simulink model "Racing_2019"  (R2017a)
settings: Solver=FixedStepDiscrete  StartTime=0.0  StopTime=Inf  FixedStep=1e-3  RelTol=1e-3  EnableMultiTasking=on
PostLoadFcn:
  | , if any(exist('dsrtsu_mdlpostloadfcn', 'file') == [2, 3, 6]), try dsrtsu_mdlpostloadfcn('Execute', bdroot); catch fprintf('Error in PostLoadFcn (dsrtsu_mdlpostloadfcn) for model "%s":\n %s\n', bdroot, lasterr); end, end,
undefined symbols (not defined in the file): Accu_Fans_Enable, Accu_Fans_ON, Accu_Fans_PWM, APPS_Bypass, APPS_Value, AUX_Error_Time, Batt_Temp_High_Threshold, Batt_Temp_Low_Threshold, BMS_Error_Time, BMS_Reset, BMS_Reset_Enable, BMS_Status_Bypass, Brake_Plausibility_Threshold, Brake_Threshold, Brakelight_Test, Braking_Torque, BSPD_State_Bypass, Buzzer, Buzzer_Silent, Buzzer_Test, Calibrate, CAN_Rx_FMEA_Enable, CAN_Status_FMEA_Enable, CAN_Tx_FMEA_Enable, Car_Reset, Car_Reset_Enable, Dash_Fan_PWM, DiscIntNeverNeededParam, DRS_Enable, DRS_PWM_OFF, DRS_PWM_ON, ED_Enable, ED_On, Eject_USB, Enable_Kill, Enable_LED_Test, Fans_Left_Enable, Fans_Left_ON, Fans_Left_PWM, Fans_Right_Enable, Fans_Right_ON, Fans_Right_PWM, I_MAX, IGBT_Temp_High_Threshold, IGBT_Temp_Low_Threshold, Inverter_CAN_Tx_Enable, Inverter_Frequency, KW_Max_Regen_Reset, KW_Max_Reset, LV_DCDC_Temp_High_Threshold, LV_DCDC_Temp_Low_Threshold, magnitude, Plausibility_Bypass, Power_Limiter_Killswitch, Power_Target_kW, Pump_Left_Enable, Pump_Left_ON, Pump_Right_Enable, Pump_Right_ON, Pump_Signal_Left ... (+13)
libraries: rtiusbflightreclib x206, simulink x153, rtican x52, powerlib_meascontrol x47, simulink_extras x17, rti1401lib_adc_type4 x6, rti1401lib_dio_type4 x3, rti1401lib_II_base x1
(part 14 of 23)

== system Racing_2019/Inverters CAN Tx ==
  note: Error = 0
  Torque Right : Inport
  Torque Left : Inport  Port=2
  10Hz Pulse : DiscretePulseGenerator  Period=100  SampleTime=0.001
  Add : Sum
  Add1 : Sum
  Add2 : Sum
  Bus Creator : BusCreator  Inputs='Mode','ID','Time'
  Bus Selector : BusSelector  OutputSignals=Mode
  Bus Selector1 : BusSelector  OutputSignals=ID,ID,ID
  Bus Selector2 : BusSelector  OutputSignals=Time,Time,Time
  Bus Selector3 : BusSelector  OutputSignals=Mode
  Bus Selector4 : BusSelector  OutputSignals=ID,ID,ID
  Bus Selector5 : BusSelector  OutputSignals=Time,Time,Time
  Bus Selector6 : BusSelector  OutputSignals=Time
  Bus Selector7 : BusSelector  OutputSignals=ID
  Bus Selector8 : BusSelector  OutputSignals=Time
  Bus Selector9 : BusSelector  OutputSignals=ID
  Constant : Constant  Value=I_MAX
  Constant1 : Constant  Value=Inverter_CAN_Tx_Enable
  Constant2 : Constant  Value=Set_Inverter_Settings
  Constant3 : Constant  Value=Set_ID
  Constant4 : Constant  Value=0
  Constant5 : Constant  Value=0
  Constant6 : Constant  Value=RPM_MAX
  Data Type Conversion{,1..2,5..6} (5 alike) : DataTypeConversion  OutDataTypeStr=double
  Data Type Conversion3 : DataTypeConversion  OutDataTypeStr=uint8
  Data Type Conversion4 : DataTypeConversion  OutDataTypeStr=uint8
  Data Type Conversion7 : DataTypeConversion  OutDataTypeStr=uint16
  Data Type Conversion8 : DataTypeConversion  OutDataTypeStr=uint16
  Data Type Conversion9 : DataTypeConversion  OutDataTypeStr=uint16
  Delay 50ms : Delay  DelayLength=50  SampleTime=0.001
  Edge Detector : powerlib_meascontrol/Logic/Edge Detector  model=Rising  ic=0  Ts=-1
      settings: SourceProductName=Simscape Power Systems  SourceProductBaseCode=PS
  Edge Detector1 : powerlib_meascontrol/Logic/Edge Detector  model=Rising  ic=0  Ts=-1
      settings: SourceProductName=Simscape Power Systems  SourceProductBaseCode=PS
  Gain_Left : Gain  Gain=-32767/1000
  Gain_Right : Gain  Gain=-32767/1000
  Inverter_LEFT_CAN_0x161 : Delay  DelayLength=1000  InitialCondition=1  ExternalReset=Level
      settings: InputPortMap=u0,r5
  Inverter_LEFT_CAN_Tx_Counter : Memory  InheritSampleTime=on
  Inverter_Left_CAN_Tx : rtican/RTICAN Transmit (TX)   Reserved1=[]  Reserved2=[]  Reserved3=[]  Reserved4=[]  SfcnMessage=[]  Msg_Struct=[]  BoardTypeNo=[]  BoardNo=[]  ChannelNo=[]  Parameters=[]  DialogFcn=[]  UnitName=[]  Revision=[]  UnitValues=[]  DSProperties=struct('RTI',struct('Version',uint32(5),'BlockType',struct('isSLSource',uint8(1),'isSLSink',uint8(1),'isHWSource',uint8(0),'isHWSink',uint8(0),'isSetup',uint8(0),'isInline',uint8(1),'isNonInline',uint8(0),'isInterrupt',uint8(0),'isChannelwise',uint8(0)),'IOBoardType','RTICAN','UnitType','MESSAGE','Identifier','TX','DialogType','MSVC','BlockSet','RTICAN','SlaveProcessor','CAN'))  RTIBlockInterface=struct('InputPortsWidth',int32([1 1 1 1 1 1 1 1 1 1]),'InputPortsActive',[1 1 1 1 1 1 1 1 1 1],'InputPortsName',{{'REGID_Mode','REGID','b1_77','b1_78','Torque_CMD','b1_200','Time','b2_77','b2_78','b2_200'}},'InputPortsDataType',{{'SS_DOUBLE','SS_DOUBLE','SS_DOUBLE','SS_DOUBLE','SS_DOUBLE','SS_DOUBLE','SS_DOUBLE','SS_DOUBLE','SS_DOUBLE','SS_DOUBLE'}},'OutputPortsWidth',int32(1),'OutputPortsActive',1,'OutputPortsName',{{['TX status']}},'DialogFcn','rtican_message_interface_gui','BlockDisplay',{{'','center'}},'IconTransparency','on','InitLevel',3,'BlockName',struct('Token',{{'Inverter_Left_CAN_Tx'}}),'SampleTime',{{0.001}},'TriggerPort',{{'none'}},'EnablePort',{{'yes'}})  RTIBlockParameters=struct('BoardTypeNo',{{1,'OFF',[]}},'BoardNo',{{1,'ON',[1 16]}},'ChannelNo',{{1,'ON',[1 2]}},'Parameters',{{struct('DataFileSupport',struct('DataFileSelectedMaster',0,'DataFileSelectedLocal',0,'DataFileName',['<no datafile support>|'],'DataFileDate','','SelectedFile',['<no file selected>']),'Options',struct('StatusSelected',1,'TimeSelected',0,'DeltaTimeSelected',0,'DelayTimeSelected',0,'DelayTimeTXCommandSelected',0,'EncodeSetUnusedBitsToOne',0,'EnableMsgLoopback',0,'TriggerPort',struct('Selected',0,'TriggerType',0),'EnablePortSelected',1,'SignalOnPortnameSelected',1,'UserCoding',struct('Selected',0,'InterfaceFile','UserEncodingFile','FcnName','UserEncodeFcn','InportSelected',0,'InportWidth',1,'OutportSelected',0,'OutportWidth',1),'TerminationMsg',struct('Selected',0,'Byte0_7','0'),'InitialMsg',struct('Selected',0,'Byte0_7','0')),'Message',struct('MsgOnBlocknameSelected',1,'MsgName','Inverter_Left_CAN_Tx','MsgIdFormat',0,'MsgId',353,'MsgLength',3,'NumSignals',10,'SampleTime',0.001,'StartTime',struct('Selected',0,'Value',9),'AutoRepeatTime',struct('Selected',0,'Value',0.1),'Timeout',struct('Selected',0,'Value',0.1),'DelayTime',struct('Selected',0,'Value',0.1),'Signal',struct('SgnName',{'REGID_Mode','REGID','b1_77','b1_78','Torque_CMD','b1_200','Time','b2_77','b2_78','b2_200'},'SgnStartBit',{0,8,8,8,8,8,16,16,16,16},'SgnLength',{8,8,8,8,16,8,8,8,8,8},'SgnType',{1,2,2,2,2,2,2,2,2,2},'ModeValue',{-1,61,77,78,144,200,61,77,78,200},'DataType',{0,0,0,0,1,0,0,0,0,0},'ByteLayout',{0,0,0,0,0,0,0,0,0,0},'Factor',{1,1,1,1,1,1,1,1,1,1},'Offset',{0,0,0,0,0,0,0,0,0,0},'SgnComment',{{''},{''},{''},{''},{''},{''},{''},{''},{''},{''}},'SgnUnit',{'','','','','','','','','',''},'Min',{0,0,0,0,0,0,0,0,0,0},'Max',{255,255,255,255,255,0,255,255,255,0},'SLDataType',{'SS_DOUBLE','SS_DOUBLE','SS_DOUBLE','SS_DOUBLE','SS_DOUBLE','SS_DOUBLE','SS_DOUBLE','SS_DOUBLE','SS_DOUBLE','SS_DOUBLE'}),'MsgIdNumFormat',1,'MsgComment',{{''}}),'Version',1.2,'general',struct('isFromLib',0)),'OFF',[]}},'GroupId',{{struct('Group',{{'RTICAN'}},'No',1,'Behavior',{{'NAMECHANGE'}},'BlockType',{{'SINK'}},'NameChangeFlag',0),'OFF',[]}},'SFcnRTICANMessage',{{struct('MsgType','TX','SFcnPortType','Scalar','MsgName','Inverter_Left_CAN_Tx','MsgIdFormat','STD','MsgId',353,'MsgLength',3,'NumSignals',10,'SampleTime',0.001,'StartTime',struct('Selected','no','Value',9),'AutoRepeatTime',struct('Selected','no','Value',0.1),'Timeout',struct('Selected','no','Value',0.1),'Signal',struct('SgnName',{'REGID_Mode','REGID','b1_77','b1_78','Torque_CMD','b1_200','Time','b2_77','b2_78','b2_200'},'SgnStartBit',{0,8,8,8,8,8,16,16,16,16},'SgnLength',{8,8,8,8,16,8,8,8,8,8},'SgnType',{'mode','mode-dependent','mode-dependent','mode-dependent','mode-dependent','mode-dependent','mode-dependent','mode-dependent','mode-dependent','mode-dependent'},'ModeValue',{-1,61,77,78,144,200,61,77,78,200},'DataType',{['unsigned int'],['unsigned int'],['unsigned int'],['unsigned int'],['signed int'],['unsigned int'],['unsigned int'],['unsigned int'],['unsigned int'],['unsigned int']},'ByteLayout',{['little endian'],['little endian'],['little endian'],['little endian'],['little endian'],['little endian'],['little endian'],['little endian'],['little endian'],['little endian']},'Factor',{1,1,1,1,1,1,1,1,1,1},'Offset',{0,0,0,0,0,0,0,0,0,0},'SLDataType',{'SS_DOUBLE','SS_DOUBLE','SS_DOUBLE','SS_DOUBLE','SS_DOUBLE','SS_DOUBLE','SS_DOUBLE','SS_DOUBLE','SS_DOUBLE','SS_DOUBLE'}),'StatusSelected','yes','TimeSelected','no','DeltaTimeSelected','no','DelayTimeSelected','no','DelayTimeTXCommandSelected','no','EncodeSetUnusedBitsToOne','no','EnableMsgLoopback','no','TriggerPort',struct('Selected','no','TriggerType',0),'EnablePortSelected','yes','UserCoding',struct('Selected','no','InterfaceFile','UserEncodingFile','FcnName','UserEncodeFcn','InportSelected','no','InportWidth',1,'OutportSelected','no','OutportWidth',1),'TerminationMsg',struct('Selected','no','Byte0','0x00','Byte1','0x00','Byte2','0x00','Byte3','0x00','Byte4','0x00','Byte5','0x00','Byte6','0x00','Byte7','0x00'),'InitialMsg',struct('Selected','no','Byte0','0x00','Byte1','0x00','Byte2','0x00','Byte3','0x00','Byte4','0x00','Byte5','0x00','Byte6','0x00','Byte7','0x00'),'BoardType','DS1','BoardNo',1,'ControllerNo',1),'OFF',[]}},'TLCFileName',{{'rtican_tx_message','OFF',[]}})  RTISFcnParameters=struct('SFcnRTICANMessage','struct','TLCFileName','char')  RTIBlockParaDefault=struct('BoardTypeNo',4302,'BoardNo',1,'ChannelNo',1,'Parameters',struct('DataFileSupport',struct('DataFileSelectedMaster',0,'DataFileSelectedLocal',0,'DataFileName','','DataFileDate','','SelectedFile',['<no file selected>']),'Options',struct('StatusSelected',1,'TimeSelected',1,'DeltaTimeSelected',1,'DelayTimeSelected',1,'DelayTimeTXCommandSelected',0,'EncodeSetUnusedBitsToOne',0,'EnableMsgLoopback',0,'TriggerPort',struct('Selected',0,'TriggerType','rising'),'EnablePortSelected',0,'SignalOnPortnameSelected',1,'UserCoding',struct('Selected',0,'InterfaceFile','UserEncodingFile','FcnName','UserEncodeFcn','InportSelected',0,'InportWidth',1,'OutportSelected',0,'OutportWidth',1),'TerminationMsg',struct('Selected',0,'Byte0_7','0'),'InitialMsg',struct('Selected',0,'Byte0_7','0')),'Message',struct('MsgOnBlocknameSelected',0,'MsgName',['TX Message'],'MsgIdFormat',0,'MsgId',100,'MsgLength',8,'NumSignals',1,'SampleTime',-1,'StartTime',struct('Selected',0,'Value',0),'AutoRepeatTime',struct('Selected',0,'Value',0.1),'Timeout',struct('Selected',0,'Value',0.1),'DelayTime',struct('Selected',0,'Value',0.1),'Signal',struct('SgnName',['TX signal'],'SgnStartBit',0,'SgnLength',8,'SgnType',0,'ModeValue',-1,'DataType',0,'SLDataType','SS_DOUBLE','ByteLayout',0,'Factor',1,'Offset',0,'Min',0,'Max',255,'SgnComment',{{}},'SgnUnit',''),'MsgIdNumFormat',0,'MsgComment',{{''}}),'Version',1.2,'general',struct('isFromLib',1)),'GroupId',struct('Group',{{'RTICAN'}},'No',1,'Behavior',{{'NAMECHANGE'}},'BlockType',{{'SINK'}},'NameChangeFlag',0),'SFcnRTICANMessage',struct('MsgType','TX','MsgName',['TX Message'],'MsgIdFormat','STD','MsgId',100,'MsgLength',2,'NumSignals',1,'SampleTime',-1,'StartTime',struct('Selected','no','Value',0),'AutoRepeatTime',struct('Selected','no','Value',0.1),'Timeout',struct('Selected','no','Value',0.1),'DelayTime',struct('Selected','no','Value',0.1),'Signal',struct('SgnName',['TX signal'],'SgnStartBit',0,'SgnLength',8,'SgnType','standard','ModeValue',-1,'DataType',['unsigned int'],'ByteLayout',['little endian'],'SLDataType','SS_DOUBLE','Factor',1,'Offset',0),'StatusSelected','yes','TimeSelected','yes','DeltaTimeSelected','yes','DelayTimeSelected','yes','EnablePortSelected','no','EnableMsgLoopback','no','DelayTimeTXCommandSelected','no','EncodeSetUnusedBitsToOne','no','UserCoding',struct('Selected','no','InterfaceFile','UserDecodingFile','FcnName','UserDecodeFcn','InportSelected','no','InportWidth',1,'OutportSelected','no','OutportWidth',1),'TerminationMsg',struct('Selected','no','Byte0','0x00','Byte1','0x00','Byte2','0x00','Byte3','0x00','Byte4','0x00','Byte5','0x00','Byte6','0x00','Byte7','0x00'),'InitialMsg',struct('Selected','no','Byte0','0x00','Byte1','0x00','Byte2','0x00','Byte3','0x00','Byte4','0x00','Byte5','0x00','Byte6','0x00','Byte7','0x00'),'TriggerPort',struct('Selected','no','TriggerType','rising'),'BoardType','DS4302','BoardNo',1,'ControllerNo',1,'SFcnPortType','Scalar'),'TLCFileName','rtican_tx_message')
      settings: AttributesFormatString=Group Id: RTICAN1\n  SourceProductName=dSPACE RTI CAN Blockset
  Inverter_RIGHT_CAN_0x162 : Delay  DelayLength=1000  InitialCondition=1  ExternalReset=Level
      settings: InputPortMap=u0,r5
  Inverter_RIGHT_CAN_Tx_Counter : Memory  InheritSampleTime=on
  Inverter_Right_CAN_Tx : rtican/RTICAN Transmit (TX)   Reserved1=[]  Reserved2=[]  Reserved3=[]  Reserved4=[]  SfcnMessage=[]  Msg_Struct=[]  BoardTypeNo=[]  BoardNo=[]  ChannelNo=[]  Parameters=[]  DialogFcn=[]  UnitName=[]  Revision=[]  UnitValues=[]  DSProperties=struct('RTI',struct('Version',uint32(5),'BlockType',struct('isSLSource',uint8(1),'isSLSink',uint8(1),'isHWSource',uint8(0),'isHWSink',uint8(0),'isSetup',uint8(0),'isInline',uint8(1),'isNonInline',uint8(0),'isInterrupt',uint8(0),'isChannelwise',uint8(0)),'IOBoardType','RTICAN','UnitType','MESSAGE','Identifier','TX','DialogType','MSVC','BlockSet','RTICAN','SlaveProcessor','CAN'))  RTIBlockInterface=struct('InputPortsWidth',int32([1 1 1 1 1 1 1 1 1 1]),'InputPortsActive',[1 1 1 1 1 1 1 1 1 1],'InputPortsName',{{'REGID_Mode','REGID','b1_77','b1_78','Torque_Value','b1_200','Time','b2_77','b2_78','b2_200'}},'InputPortsDataType',{{'SS_DOUBLE','SS_DOUBLE','SS_DOUBLE','SS_DOUBLE','SS_DOUBLE','SS_DOUBLE','SS_DOUBLE','SS_DOUBLE','SS_DOUBLE','SS_DOUBLE'}},'OutputPortsWidth',int32(1),'OutputPortsActive',1,'OutputPortsName',{{['TX status']}},'DialogFcn','rtican_message_interface_gui','BlockDisplay',{{'','center'}},'IconTransparency','on','InitLevel',3,'BlockName',struct('Token',{{'Inverter_Right_CAN_Tx'}}),'SampleTime',{{0.001}},'TriggerPort',{{'none'}},'EnablePort',{{'yes'}})  RTIBlockParameters=struct('BoardTypeNo',{{1,'OFF',[]}},'BoardNo',{{1,'ON',[1 16]}},'ChannelNo',{{2,'ON',[1 2]}},'Parameters',{{struct('DataFileSupport',struct('DataFileSelectedMaster',0,'DataFileSelectedLocal',0,'DataFileName',['<no datafile support>|'],'DataFileDate','','SelectedFile',['<no file selected>']),'Options',struct('StatusSelected',1,'TimeSelected',0,'DeltaTimeSelected',0,'DelayTimeSelected',0,'DelayTimeTXCommandSelected',0,'EncodeSetUnusedBitsToOne',0,'EnableMsgLoopback',0,'TriggerPort',struct('Selected',0,'TriggerType',0),'EnablePortSelected',1,'SignalOnPortnameSelected',1,'UserCoding',struct('Selected',0,'InterfaceFile','UserEncodingFile','FcnName','UserEncodeFcn','InportSelected',0,'InportWidth',1,'OutportSelected',0,'OutportWidth',1),'TerminationMsg',struct('Selected',0,'Byte0_7','0'),'InitialMsg',struct('Selected',0,'Byte0_7','0')),'Message',struct('MsgOnBlocknameSelected',1,'MsgName','Inverter_Right_CAN_Tx','MsgIdFormat',0,'MsgId',354,'MsgLength',3,'NumSignals',10,'SampleTime',0.001,'StartTime',struct('Selected',0,'Value',5),'AutoRepeatTime',struct('Selected',0,'Value',0.1),'Timeout',struct('Selected',0,'Value',0.1),'DelayTime',struct('Selected',0,'Value',0.1),'Signal',struct('SgnName',{'REGID_Mode','REGID','b1_77','b1_78','Torque_Value','b1_200','Time','b2_77','b2_78','b2_200'},'SgnStartBit',{0,8,8,8,8,8,16,16,16,16},'SgnLength',{8,8,8,8,16,8,8,8,8,8},'SgnType',{1,2,2,2,2,2,2,2,2,2},'ModeValue',{-1,61,77,78,144,200,61,77,78,200},'DataType',{0,0,0,0,1,0,0,0,0,0},'ByteLayout',{0,0,0,0,0,0,0,0,0,0},'Factor',{1,1,1,1,1,1,1,1,1,1},'Offset',{0,0,0,0,0,0,0,0,0,0},'SgnComment',{{''},{''},{''},{''},{''},{''},{''},{''},{''},{''}},'SgnUnit',{'','','','','','','','','',''},'Min',{0,0,0,0,0,0,0,0,0,0},'Max',{255,255,255,255,255,0,255,255,255,0},'SLDataType',{'SS_DOUBLE','SS_DOUBLE','SS_DOUBLE','SS_DOUBLE','SS_DOUBLE','SS_DOUBLE','SS_DOUBLE','SS_DOUBLE','SS_DOUBLE','SS_DOUBLE'}),'MsgIdNumFormat',1,'MsgComment',{{''}}),'Version',1.2,'general',struct('isFromLib',0)),'OFF',[]}},'GroupId',{{struct('Group',{{'RTICAN'}},'No',2,'Behavior',{{'NAMECHANGE'}},'BlockType',{{'SINK'}},'NameChangeFlag',0),'OFF',[]}},'SFcnRTICANMessage',{{struct('MsgType','TX','SFcnPortType','Scalar','MsgName','Inverter_Right_CAN_Tx','MsgIdFormat','STD','MsgId',354,'MsgLength',3,'NumSignals',10,'SampleTime',0.001,'StartTime',struct('Selected','no','Value',5),'AutoRepeatTime',struct('Selected','no','Value',0.1),'Timeout',struct('Selected','no','Value',0.1),'Signal',struct('SgnName',{'REGID_Mode','REGID','b1_77','b1_78','Torque_Value','b1_200','Time','b2_77','b2_78','b2_200'},'SgnStartBit',{0,8,8,8,8,8,16,16,16,16},'SgnLength',{8,8,8,8,16,8,8,8,8,8},'SgnType',{'mode','mode-dependent','mode-dependent','mode-dependent','mode-dependent','mode-dependent','mode-dependent','mode-dependent','mode-dependent','mode-dependent'},'ModeValue',{-1,61,77,78,144,200,61,77,78,200},'DataType',{['unsigned int'],['unsigned int'],['unsigned int'],['unsigned int'],['signed int'],['unsigned int'],['unsigned int'],['unsigned int'],['unsigned int'],['unsigned int']},'ByteLayout',{['little endian'],['little endian'],['little endian'],['little endian'],['little endian'],['little endian'],['little endian'],['little endian'],['little endian'],['little endian']},'Factor',{1,1,1,1,1,1,1,1,1,1},'Offset',{0,0,0,0,0,0,0,0,0,0},'SLDataType',{'SS_DOUBLE','SS_DOUBLE','SS_DOUBLE','SS_DOUBLE','SS_DOUBLE','SS_DOUBLE','SS_DOUBLE','SS_DOUBLE','SS_DOUBLE','SS_DOUBLE'}),'StatusSelected','yes','TimeSelected','no','DeltaTimeSelected','no','DelayTimeSelected','no','DelayTimeTXCommandSelected','no','EncodeSetUnusedBitsToOne','no','EnableMsgLoopback','no','TriggerPort',struct('Selected','no','TriggerType',0),'EnablePortSelected','yes','UserCoding',struct('Selected','no','InterfaceFile','UserEncodingFile','FcnName','UserEncodeFcn','InportSelected','no','InportWidth',1,'OutportSelected','no','OutportWidth',1),'TerminationMsg',struct('Selected','no','Byte0','0x00','Byte1','0x00','Byte2','0x00','Byte3','0x00','Byte4','0x00','Byte5','0x00','Byte6','0x00','Byte7','0x00'),'InitialMsg',struct('Selected','no','Byte0','0x00','Byte1','0x00','Byte2','0x00','Byte3','0x00','Byte4','0x00','Byte5','0x00','Byte6','0x00','Byte7','0x00'),'BoardType','DS1','BoardNo',1,'ControllerNo',2),'OFF',[]}},'TLCFileName',{{'rtican_tx_message','OFF',[]}})  RTISFcnParameters=struct('SFcnRTICANMessage','struct','TLCFileName','char')  RTIBlockParaDefault=struct('BoardTypeNo',4302,'BoardNo',1,'ChannelNo',1,'Parameters',struct('DataFileSupport',struct('DataFileSelectedMaster',0,'DataFileSelectedLocal',0,'DataFileName','','DataFileDate','','SelectedFile',['<no file selected>']),'Options',struct('StatusSelected',1,'TimeSelected',1,'DeltaTimeSelected',1,'DelayTimeSelected',1,'DelayTimeTXCommandSelected',0,'EncodeSetUnusedBitsToOne',0,'EnableMsgLoopback',0,'TriggerPort',struct('Selected',0,'TriggerType','rising'),'EnablePortSelected',0,'SignalOnPortnameSelected',1,'UserCoding',struct('Selected',0,'InterfaceFile','UserEncodingFile','FcnName','UserEncodeFcn','InportSelected',0,'InportWidth',1,'OutportSelected',0,'OutportWidth',1),'TerminationMsg',struct('Selected',0,'Byte0_7','0'),'InitialMsg',struct('Selected',0,'Byte0_7','0')),'Message',struct('MsgOnBlocknameSelected',0,'MsgName',['TX Message'],'MsgIdFormat',0,'MsgId',100,'MsgLength',8,'NumSignals',1,'SampleTime',-1,'StartTime',struct('Selected',0,'Value',0),'AutoRepeatTime',struct('Selected',0,'Value',0.1),'Timeout',struct('Selected',0,'Value',0.1),'DelayTime',struct('Selected',0,'Value',0.1),'Signal',struct('SgnName',['TX signal'],'SgnStartBit',0,'SgnLength',8,'SgnType',0,'ModeValue',-1,'DataType',0,'SLDataType','SS_DOUBLE','ByteLayout',0,'Factor',1,'Offset',0,'Min',0,'Max',255,'SgnComment',{{}},'SgnUnit',''),'MsgIdNumFormat',0,'MsgComment',{{''}}),'Version',1.2,'general',struct('isFromLib',1)),'GroupId',struct('Group',{{'RTICAN'}},'No',1,'Behavior',{{'NAMECHANGE'}},'BlockType',{{'SINK'}},'NameChangeFlag',0),'SFcnRTICANMessage',struct('MsgType','TX','MsgName',['TX Message'],'MsgIdFormat','STD','MsgId',100,'MsgLength',2,'NumSignals',1,'SampleTime',-1,'StartTime',struct('Selected','no','Value',0),'AutoRepeatTime',struct('Selected','no','Value',0.1),'Timeout',struct('Selected','no','Value',0.1),'DelayTime',struct('Selected','no','Value',0.1),'Signal',struct('SgnName',['TX signal'],'SgnStartBit',0,'SgnLength',8,'SgnType','standard','ModeValue',-1,'DataType',['unsigned int'],'ByteLayout',['little endian'],'SLDataType','SS_DOUBLE','Factor',1,'Offset',0),'StatusSelected','yes','TimeSelected','yes','DeltaTimeSelected','yes','DelayTimeSelected','yes','EnablePortSelected','no','EnableMsgLoopback','no','DelayTimeTXCommandSelected','no','EncodeSetUnusedBitsToOne','no','UserCoding',struct('Selected','no','InterfaceFile','UserDecodingFile','FcnName','UserDecodeFcn','InportSelected','no','InportWidth',1,'OutportSelected','no','OutportWidth',1),'TerminationMsg',struct('Selected','no','Byte0','0x00','Byte1','0x00','Byte2','0x00','Byte3','0x00','Byte4','0x00','Byte5','0x00','Byte6','0x00','Byte7','0x00'),'InitialMsg',struct('Selected','no','Byte0','0x00','Byte1','0x00','Byte2','0x00','Byte3','0x00','Byte4','0x00','Byte5','0x00','Byte6','0x00','Byte7','0x00'),'TriggerPort',struct('Selected','no','TriggerType','rising'),'BoardType','DS4302','BoardNo',1,'ControllerNo',1,'SFcnPortType','Scalar'),'TLCFileName','rtican_tx_message')
      settings: AttributesFormatString=Group Id: RTICAN2\n  SourceProductName=dSPACE RTI CAN Blockset
  Inverters CAN Send : MATLAB Function  TreatAsAtomicUnit=on
  Logical Operator : Logic  Inputs=3  AllPortsSameDT=off  OutDataTypeStr=boolean
  Logical Operator1 : Logic  Operator=NOT  AllPortsSameDT=off  OutDataTypeStr=boolean
  Logical Operator2 : Logic  AllPortsSameDT=off  OutDataTypeStr=boolean
  Memory : Memory  X0=-14
  Switch : Switch  Criteria=u2 > Threshold
  Switch1 : Switch  Criteria=u2 > Threshold
  Torque AND : Logic  AllPortsSameDT=off  OutDataTypeStr=boolean
  Torque Mode : simulink/Logic and Bit Operations/Compare To Constant  relop===  const=144  OutDataTypeStr=boolean
  USB_Torque_Left : rtiusbflightreclib/USB_FLIGHT_REC_BL1  VarName=Torque_Left  DataType=UInt16  SampleTime=-1  TLCFileName=rtiusbflightrecwrite  Reserved1=[]  Reserved2=[]  Reserved3=[]  Reserved4=[]  DSProperties=struct('RTI',struct('Version',uint32(3),'BlockType',struct('isSLSource',uint8(0),'isSLSink',uint8(1),'isHWSource',uint8(0),'isHWSink',uint8(0),'isSetup',uint8(0),'isInline',uint8(1),'isNonInline',uint8(0),'isInterrupt',uint8(0),'isChannelwise',uint8(0)),'IOBoardType',{{'DSUSB','FLIGHTREC'}},'UnitType','FLIGHTREC','Identifier','WRITE','DialogType','SL','BlockSet','RTIUSBFLIGHTREC','SlaveProcessor','NONE'))  RTIBlockInterface=struct('InputPortsActive',1,'InputPortsWidth',int32(1),'InputPortsDataType',{{'SS_UINT16'}},'BlockDisplay',{{['Write to\nUSB Flight Recorder'],'center'}},'IconTransparency','off','InitLevel',3,'BlockName',struct('Token',{{'USB_FLIGHT_REC_BL1'}}),'MaskDescription',['Write input to the Flight Recorder. Recorded data can be referenced by the specified variable.'],'SampleTime',{{-1}})  RTIBlockParameters=struct('VarName',{{'Torque_Left','OFF',[]}},'DataType',{{'UInt16','OFF',[]}},'SampleTime',{{-1,'OFF',[]}},'TLCFileName',{{'rtiusbflightrecwrite','OFF',[]}})  RTISFcnParameters=struct('VarName','char','DataType','char','SampleTime','double','TLCFileName','char')  RTIBlockParaDefault=struct('VarName','Var1','DataType','Single','SampleTime',-1,'TLCFileName','rtiusbflightrecwrite')
      settings: SourceProductName=dSPACE RTI USB Flight Rec Blockset
  USB_Torque_Right : rtiusbflightreclib/USB_FLIGHT_REC_BL1  VarName=Torque_Right  DataType=UInt16  SampleTime=-1  TLCFileName=rtiusbflightrecwrite  Reserved1=[]  Reserved2=[]  Reserved3=[]  Reserved4=[]  DSProperties=struct('RTI',struct('Version',uint32(3),'BlockType',struct('isSLSource',uint8(0),'isSLSink',uint8(1),'isHWSource',uint8(0),'isHWSink',uint8(0),'isSetup',uint8(0),'isInline',uint8(1),'isNonInline',uint8(0),'isInterrupt',uint8(0),'isChannelwise',uint8(0)),'IOBoardType',{{'DSUSB','FLIGHTREC'}},'UnitType','FLIGHTREC','Identifier','WRITE','DialogType','SL','BlockSet','RTIUSBFLIGHTREC','SlaveProcessor','NONE'))  RTIBlockInterface=struct('InputPortsActive',1,'InputPortsWidth',int32(1),'InputPortsDataType',{{'SS_UINT16'}},'BlockDisplay',{{['Write to\nUSB Flight Recorder'],'center'}},'IconTransparency','off','InitLevel',3,'BlockName',struct('Token',{{'USB_FLIGHT_REC_BL1'}}),'MaskDescription',['Write input to the Flight Recorder. Recorded data can be referenced by the specified variable.'],'SampleTime',{{-1}})  RTIBlockParameters=struct('VarName',{{'Torque_Right','OFF',[]}},'DataType',{{'UInt16','OFF',[]}},'SampleTime',{{-1,'OFF',[]}},'TLCFileName',{{'rtiusbflightrecwrite','OFF',[]}})  RTISFcnParameters=struct('VarName','char','DataType','char','SampleTime','double','TLCFileName','char')  RTIBlockParaDefault=struct('VarName','Var1','DataType','Single','SampleTime',-1,'TLCFileName','rtiusbflightrecwrite')
      settings: SourceProductName=dSPACE RTI USB Flight Rec Blockset
  "Torque CAN " : Outport
  wires:
  Inverters CAN Send/1(Mode) -> Data Type Conversion/1
  Inverters CAN Send/2(ID) -> Data Type Conversion1/1
  Inverters CAN Send/3(Time) -> Data Type Conversion2/1
  Data Type Conversion/1 -> Torque Mode/1, Bus Creator/1  "Mode"
  Data Type Conversion1/1 -> Bus Creator/2  "ID"
  Data Type Conversion2/1 -> Bus Creator/3  "Time"
  Bus Selector/1 -> Inverter_Right_CAN_Tx/1  "<Mode>"
  Bus Selector1/1 -> Inverter_Right_CAN_Tx/2  "<ID>"
  Bus Selector1/2 -> Inverter_Right_CAN_Tx/3  "<ID>"
  Bus Selector1/3 -> Inverter_Right_CAN_Tx/4  "<ID>"
  Bus Selector2/1 -> Inverter_Right_CAN_Tx/7  "<Time>"
  Bus Selector2/2 -> Inverter_Right_CAN_Tx/8  "<Time>"
  Bus Selector2/3 -> Inverter_Right_CAN_Tx/9  "<Time>"
  Bus Selector4/3 -> Inverter_Left_CAN_Tx/4  "<ID>"
  Bus Selector5/3 -> Inverter_Left_CAN_Tx/9  "<Time>"
  Bus Selector3/1 -> Inverter_Left_CAN_Tx/1  "<Mode>"
  Bus Creator/1 -> Bus Selector7/1, Bus Selector/1, Bus Selector1/1, Bus Selector2/1, Bus Selector6/1, Bus Selector9/1, Bus Selector8/1, Bus Selector5/1, Bus Selector4/1, Bus Selector3/1
  Bus Selector4/1 -> Inverter_Left_CAN_Tx/2  "<ID>"
  Bus Selector5/1 -> Inverter_Left_CAN_Tx/7  "<Time>"
  Bus Selector4/2 -> Inverter_Left_CAN_Tx/3  "<ID>"
  Bus Selector5/2 -> Inverter_Left_CAN_Tx/8  "<Time>"
  Constant/1 -> Inverters CAN Send/2(Icont)
  Torque Mode/1 -> Logical Operator/1, Switch/2, Logical Operator1/1, Switch/1
  Delay 50ms/1 -> Switch/3
  Switch/1 -> Torque AND/2
  Constant1/1 -> Torque AND/1
  10Hz Pulse/1 -> Logical Operator2/1, Delay 50ms/1
  Logical Operator2/1 -> Data Type Conversion7/1
  Add/1 -> Memory/1
  Memory/1 -> Switch1/3, Inverters CAN Send/1(i)
  Switch1/1 -> Add/2
  Constant2/1 -> Switch1/2
  Constant3/1 -> Switch1/1
  Logical Operator/1 -> "Torque CAN "/1
  Edge Detector/1 -> Data Type Conversion3/1
  Inverter_LEFT_CAN_Tx_Counter/1 -> Add1/2
  Data Type Conversion3/1 -> Add1/1
  Add1/1 -> Inverter_LEFT_CAN_Tx_Counter/1
  Inverter_Left_CAN_Tx/1 -> Inverter_LEFT_CAN_0x161/2, Edge Detector/1
  Add2/1 -> Inverter_RIGHT_CAN_Tx_Counter/1
  Inverter_RIGHT_CAN_Tx_Counter/1 -> Add2/2
  Edge Detector1/1 -> Data Type Conversion4/1
  Data Type Conversion4/1 -> Add2/1
  Inverter_Right_CAN_Tx/1 -> Inverter_RIGHT_CAN_0x162/2, Edge Detector1/1
  Torque AND/1 -> Inverter_Left_CAN_Tx/Enable, Inverter_Right_CAN_Tx/Enable
  Data Type Conversion5/1 -> Inverter_Right_CAN_Tx/5
  Data Type Conversion6/1 -> Inverter_Left_CAN_Tx/5
  Logical Operator1/1 -> Logical Operator2/2
  Data Type Conversion7/1 -> Add/1
  Constant4/1 -> Inverter_RIGHT_CAN_0x162/1
  Constant5/1 -> Inverter_LEFT_CAN_0x161/1
  Inverter_RIGHT_CAN_0x162/1 -> Logical Operator/2
  Inverter_LEFT_CAN_0x161/1 -> Logical Operator/3
  Torque Left/1 -> Gain_Left/1, Data Type Conversion9/1
  Torque Right/1 -> Data Type Conversion8/1, Gain_Right/1
  Gain_Right/1 -> Data Type Conversion5/1
  Gain_Left/1 -> Data Type Conversion6/1
  Data Type Conversion8/1 -> USB_Torque_Right/1
  Data Type Conversion9/1 -> USB_Torque_Left/1
  Constant6/1 -> Inverters CAN Send/3(RPMmax)
  Bus Selector6/1 -> Inverter_Right_CAN_Tx/10  "<Time>"
  Bus Selector7/1 -> Inverter_Right_CAN_Tx/6  "<ID>"
  Bus Selector8/1 -> Inverter_Left_CAN_Tx/10  "<Time>"
  Bus Selector9/1 -> Inverter_Left_CAN_Tx/6  "<ID>"

== system Racing_2019/RTI Data ==
  RTI Data Store : Subsystem  Tag="struct('public',struct('sub',struct('name',{{'Racing_2019'}},'data',{{struct('TH',struct('thTaskInfo',struct('taskType',{'TIMER','HWINT','TMRINT','SWINT','GLINT'},'tasksNumOf',{5,0,0,0,0},'srcIds',{{'TIMERA','TIMERA2','TIMERA3','TIMERA4','TIMERA5'},{},{},{},{}},'taskNames',{{['Timer Task 1'],['Timer Task 2'],['Timer Task 3'],['Timer Task 4'],['Timer Task 5']},{},{},{},{}})),'th_tc',struct('dataType',{'TASK','TASK','TASK','TASK','TASK'},'taskGroupId',{'','','','',''},'taskGroupList',{{},{},{},{},{}},'taskSchedulingPolicy',{'FCFS','FCFS','FCFS','FCFS','FCFS'},'taskType',{'TIMER','TIMER','TIMER','TIMER','TIMER'},'blkh',{-1,-1,-1,-1,-1},'srcId',{'TIMERA','TIMERA2','TIMERA3','TIMERA4','TIMERA5'},'srcSgnName',{['Timer A interrupt'],['Timer Task 1'],['Timer Task 1'],['Timer Task 1'],['Timer Task 1']},'srcCpuName',{'','','','',''},'taskName',{['Timer Task 1  [0.001] s'],['Timer Task 2  [0.01] s'],['Timer Task 3  [0.1] s'],['Timer Task 4  [0.2] s'],['Timer Task 5  [1] s']},'taskNameDisplayExt',{'','','','',''},'smplTime',{0.001,0.01,0.1,0.2,1},'smplTimeOffs',{0,0,0,0,0},'hasFixedPriority',{0,0,0,0,0},'priority',{1,2,3,4,5},'hasFixedOvc',{0,0,0,0,0},'ovcType',{1,1,1,1,1},'ovcMax',{1,1,1,1,1}),'tc_th',struct('dataType',{'TASK','TASK','TASK','TASK','TASK'},'taskGroupId',{'','','','',''},'taskGroupList',{{},{},{},{},{}},'taskSchedulingPolicy',{'FCFS','FCFS','FCFS','FCFS','FCFS'},'taskType',{'TIMER','TIMER','TIMER','TIMER','TIMER'},'blkh',{-1,-1,-1,-1,-1},'srcId',{'TIMERA','TIMERA2','TIMERA3','TIMERA4','TIMERA5'},'srcSgnName',{['Timer A interrupt'],['Timer Task 1'],['Timer Task 1'],['Timer Task 1'],['Timer Task 1']},'srcCpuName',{'','','','',''},'taskName',{['Timer Task 1  [0.001] s'],['Timer Task 2  [0.01] s'],['Timer Task 3  [0.1] s'],['Timer Task 4  [0.2] s'],['Timer Task 5  [1] s']},'taskNameDisplayExt',{'','','','',''},'smplTime',{0.001,0.01,0.1,0.2,1},'smplTimeOffs',{0,0,0,0,0},'hasFixedPriority',{0,0,0,0,0},'priority',{1,2,3,4,5},'hasFixedOvc',{0,0,0,0,0},'ovcType',{1,1,1,1,1},'ovcMax',{1,1,1,1,1}))}})),'private',struct('version',struct('dsVer',uint32(2)),'access',struct('modified',['22-Feb-2020 11:57:05'],'type','Model','isPerm',1)))"  mask(RTI_DATA_STORE){}
      mask help:
      | RTI Data Store Block. This block is used by RTI to store internal model dependent data. Deleting this block will result in data loss.
      |
      | NEVER DELETE, COPY, OR MODIFY THIS BLOCK!
      mask Help:
      | RTI Data Store Block. This block is used by RTI to store internal model dependent data. Deleting this block will result in data loss.
      | 
      | NEVER DELETE, COPY, OR MODIFY THIS BLOCK!
      mask Display: text(0.5, 0.5, ' ', 'HorizontalAlignment', 'center');

== system Racing_2019/Regen Handler ==
  APPS : Inport
  Battery Max Temp : Inport  Port=2
  RPM Max : Inport  Port=3
  RPM Min : Inport  Port=4
  VDC : Inport  Port=5
  IDC : Inport  Port=6
  5Hz to 1kHz : RateTransition  OutPortSampleTime=0.001
  Constant : Constant  Value=Regen_Enable
  Data Type Conversion : DataTypeConversion  OutDataTypeStr=uint8
  No Boom : simulink/Logic and Bit Operations/Compare To Constant  relop=<=  const=352  OutDataTypeStr=boolean
  No Cheetah : simulink/Logic and Bit Operations/Compare To Constant  relop=<=  const=3000  OutDataTypeStr=boolean
  No Fire : simulink/Logic and Bit Operations/Compare To Constant  relop=<=  const=55  OutDataTypeStr=boolean
  No Gas : simulink/Logic and Bit Operations/Compare To Zero  relop===  OutDataTypeStr=boolean
  No Turtle : simulink/Logic and Bit Operations/Compare To Constant  relop=>=  const=600  OutDataTypeStr=boolean
  Regen AND : Logic  Inputs=7  AllPortsSameDT=off  OutDataTypeStr=boolean
  Terminator : Terminator
  USB_Regen_Enable : rtiusbflightreclib/USB_FLIGHT_REC_BL1  VarName=Regen_AND  DataType=UInt8  SampleTime=-1  TLCFileName=rtiusbflightrecwrite  Reserved1=[]  Reserved2=[]  Reserved3=[]  Reserved4=[]  DSProperties=struct('RTI',struct('Version',uint32(3),'BlockType',struct('isSLSource',uint8(0),'isSLSink',uint8(1),'isHWSource',uint8(0),'isHWSink',uint8(0),'isSetup',uint8(0),'isInline',uint8(1),'isNonInline',uint8(0),'isInterrupt',uint8(0),'isChannelwise',uint8(0)),'IOBoardType',{{'DSUSB','FLIGHTREC'}},'UnitType','FLIGHTREC','Identifier','WRITE','DialogType','SL','BlockSet','RTIUSBFLIGHTREC','SlaveProcessor','NONE'))  RTIBlockInterface=struct('InputPortsActive',1,'InputPortsWidth',int32(1),'InputPortsDataType',{{'SS_UINT8'}},'BlockDisplay',{{['Write to\nUSB Flight Recorder'],'center'}},'IconTransparency','off','InitLevel',3,'BlockName',struct('Token',{{'USB_FLIGHT_REC_BL1'}}),'MaskDescription',['Write input to the Flight Recorder. Recorded data can be referenced by the specified variable.'],'SampleTime',{{-1}})  RTIBlockParameters=struct('VarName',{{'Regen_AND','OFF',[]}},'DataType',{{'UInt8','OFF',[]}},'SampleTime',{{-1,'OFF',[]}},'TLCFileName',{{'rtiusbflightrecwrite','OFF',[]}})  RTISFcnParameters=struct('VarName','char','DataType','char','SampleTime','double','TLCFileName','char')  RTIBlockParaDefault=struct('VarName','Var1','DataType','Single','SampleTime',-1,'TLCFileName','rtiusbflightrecwrite')
      settings: SourceProductName=dSPACE RTI USB Flight Rec Blockset
  Regen Enable : Outport
  wires:
  APPS/1 -> No Gas/1
  Battery Max Temp/1 -> 5Hz to 1kHz/1
  RPM Max/1 -> No Cheetah/1
  RPM Min/1 -> No Turtle/1
  VDC/1 -> No Boom/1
  No Gas/1 -> Regen AND/1
  Constant/1 -> Regen AND/7, Regen AND/6
  No Fire/1 -> Regen AND/2
  No Cheetah/1 -> Regen AND/3
  No Turtle/1 -> Regen AND/4
  No Boom/1 -> Regen AND/5
  Regen AND/1 -> Data Type Conversion/1, Regen Enable/1
  Data Type Conversion/1 -> USB_Regen_Enable/1
  5Hz to 1kHz/1 -> No Fire/1
  IDC/1 -> Terminator/1

== system Racing_2019/Sensor Error Check ==
  "Brake " : Inport
  APPS1 : Inport  Port=2
  APPS2 : Inport  Port=3
  Steering : Inport  Port=4
  APPS1_Error_OR : Logic  Operator=OR  AllPortsSameDT=off  OutDataTypeStr=boolean
  APPS2_Error_OR : Logic  Operator=OR  AllPortsSameDT=off  OutDataTypeStr=boolean
  APPS_NotAgree_Error_OR : Logic  Operator=OR  AllPortsSameDT=off  OutDataTypeStr=boolean
  Brake_Error_OR : Logic  Operator=OR  AllPortsSameDT=off  OutDataTypeStr=boolean
  Compare To Constant10 : simulink/Logic and Bit Operations/Compare To Constant  relop=<  const=10  OutDataTypeStr=boolean
  Compare To Constant11 : simulink/Logic and Bit Operations/Compare To Constant  relop=>  const=2000  OutDataTypeStr=boolean
  Compare To Constant12 : simulink/Logic and Bit Operations/Compare To Constant  relop=<  const=10  OutDataTypeStr=boolean
  Compare To Constant13 : simulink/Logic and Bit Operations/Compare To Constant  relop=>  const=4000  OutDataTypeStr=boolean
  Compare To Constant4 : simulink/Logic and Bit Operations/Compare To Constant  relop=<  const=100  OutDataTypeStr=boolean
  Compare To Constant5 : simulink/Logic and Bit Operations/Compare To Constant  relop=>  const=5000  OutDataTypeStr=boolean
  Compare To Constant6 : simulink/Logic and Bit Operations/Compare To Constant  relop=<  const=50  OutDataTypeStr=boolean
  Compare To Constant7 : simulink/Logic and Bit Operations/Compare To Constant  relop=>  const=5000  OutDataTypeStr=boolean
  Compare To Constant8 : simulink/Logic and Bit Operations/Compare To Constant  relop=<  const=50  OutDataTypeStr=boolean
  Compare To Constant9 : simulink/Logic and Bit Operations/Compare To Constant  relop=>  const=5000  OutDataTypeStr=boolean
  Counter : Subsystem
  Counter1 : Subsystem
  Counter2 : Subsystem
  Counter3 : Subsystem
  Counter4 : Subsystem
  Counter5 : Subsystem
  Data Type Conversion : DataTypeConversion  OutDataTypeStr=uint16
  Resettable Delay 50ms : Delay  DelayLength=50  ExternalReset=Falling
      settings: InputPortMap=u0,r5
  Sensor_Error_OR : Logic  Operator=OR  Inputs=5  AllPortsSameDT=off  OutDataTypeStr=boolean
  Steering_Error_OR : Logic  Operator=OR  AllPortsSameDT=off  OutDataTypeStr=boolean
  Substract : Sum  Inputs=-+
  USB_FLIGHT_REC_Sensor_Error : rtiusbflightreclib/USB_FLIGHT_REC_BL1  VarName=Sensor_Error  DataType=UInt16  SampleTime=-1  TLCFileName=rtiusbflightrecwrite  Reserved1=[]  Reserved2=[]  Reserved3=[]  Reserved4=[]  DSProperties=struct('RTI',struct('Version',uint32(3),'BlockType',struct('isSLSource',uint8(0),'isSLSink',uint8(1),'isHWSource',uint8(0),'isHWSink',uint8(0),'isSetup',uint8(0),'isInline',uint8(1),'isNonInline',uint8(0),'isInterrupt',uint8(0),'isChannelwise',uint8(0)),'IOBoardType',{{'DSUSB','FLIGHTREC'}},'UnitType','FLIGHTREC','Identifier','WRITE','DialogType','SL','BlockSet','RTIUSBFLIGHTREC','SlaveProcessor','NONE'))  RTIBlockInterface=struct('InputPortsActive',1,'InputPortsWidth',int32(1),'InputPortsDataType',{{'SS_UINT16'}},'BlockDisplay',{{['Write to\nUSB Flight Recorder'],'center'}},'IconTransparency','off','InitLevel',3,'BlockName',struct('Token',{{'USB_FLIGHT_REC_BL1'}}),'MaskDescription',['Write input to the Flight Recorder. Recorded data can be referenced by the specified variable.'],'SampleTime',{{-1}})  RTIBlockParameters=struct('VarName',{{'Sensor_Error','OFF',[]}},'DataType',{{'UInt16','OFF',[]}},'SampleTime',{{-1,'OFF',[]}},'TLCFileName',{{'rtiusbflightrecwrite','OFF',[]}})  RTISFcnParameters=struct('VarName','char','DataType','char','SampleTime','double','TLCFileName','char')  RTIBlockParaDefault=struct('VarName','Var1','DataType','Single','SampleTime',-1,'TLCFileName','rtiusbflightrecwrite')
      settings: SourceProductName=dSPACE RTI USB Flight Rec Blockset
  Sensor Error : Outport
  wires:
  Data Type Conversion/1 -> USB_FLIGHT_REC_Sensor_Error/1
  Compare To Constant6/1 -> APPS1_Error_OR/1
  Compare To Constant10/1 -> APPS_NotAgree_Error_OR/1
  Sensor_Error_OR/1 -> Resettable Delay 50ms/2, Resettable Delay 50ms/1
  Compare To Constant13/1 -> Steering_Error_OR/2
  Compare To Constant5/1 -> Brake_Error_OR/2
  Compare To Constant4/1 -> Brake_Error_OR/1
  APPS2_Error_OR/1 -> Counter3/1(In1), Sensor_Error_OR/4
  Substract/1 -> Compare To Constant11/1, Compare To Constant10/1
  APPS1_Error_OR/1 -> Counter1/1(In1), Sensor_Error_OR/2
  Brake_Error_OR/1 -> Counter/1(In1), Sensor_Error_OR/1
  Resettable Delay 50ms/1 -> Data Type Conversion/1, Sensor Error/1, Counter5/1(In1)
  Compare To Constant8/1 -> APPS2_Error_OR/1
  Compare To Constant7/1 -> APPS1_Error_OR/2
  Compare To Constant11/1 -> APPS_NotAgree_Error_OR/2
  Compare To Constant9/1 -> APPS2_Error_OR/2
  Compare To Constant12/1 -> Steering_Error_OR/1
  Steering/1 -> Compare To Constant13/1, Compare To Constant12/1
  "Brake "/1 -> Compare To Constant4/1, Compare To Constant5/1
  APPS2/1 -> Compare To Constant9/1, Compare To Constant8/1, Substract/2
  APPS1/1 -> Compare To Constant7/1, Compare To Constant6/1, Substract/1
  Steering_Error_OR/1 -> Sensor_Error_OR/5, Counter4/1(In1)
  APPS_NotAgree_Error_OR/1 -> Sensor_Error_OR/3, Counter2/1(In1)

== system Racing_2019/The Journey of Torque ==
  "IDC " : Inport
  RPM Max : Inport  Port=2
  Irms Left : Inport  Port=3
  Irms Right : Inport  Port=4
  APPS : Inport  Port=5
  Steering : Inport  Port=6
  Differential Toggle : Inport  Port=7
  "Regen Enable " : Inport  Port=8
  Bus Creator : BusCreator  Inputs='IDC','RPM Max','Irms Left','Irms Right','APPS','Steering','Differential Toggle','Regen Enable'
  Bus Selector : BusSelector  OutputSignals=IDC,RPM Max,Irms Left,Irms Right,APPS
  Bus Selector1 : BusSelector  OutputSignals=Steering,Differential Toggle
  Bus Selector2 : BusSelector  OutputSignals=IDC,Regen Enable
  Bus Selector3 : BusSelector  OutputSignals=Regen Enable
  Electronic Differential : Subsystem
  Enable Torque : Constant
  Left Torque Switch : Switch  Criteria=u2 > Threshold
  Power Limiter v3 (open-loop) : Subsystem
  Power Target in kW1 : Constant  Value=Power_Target_kW
  Regen : Subsystem
  Regen Torque : Constant  Value=0
  Right Torque Switch : Switch  Criteria=u2 > Threshold
  Switch2 : Switch  Criteria=u2 > Threshold
  "Torque Right " : Outport
  Torque Left : Outport  Port=2
  wires:
  Right Torque Switch/1 -> "Torque Right "/1
  Left Torque Switch/1 -> Torque Left/1
  Switch2/1 -> Right Torque Switch/2, Left Torque Switch/2
  Enable Torque/1 -> Switch2/3
  Regen Torque/1 -> Switch2/1
  "IDC "/1 -> Bus Creator/1  "IDC"
  RPM Max/1 -> Bus Creator/2  "RPM Max"
  Irms Left/1 -> Bus Creator/3  "Irms Left"
  Irms Right/1 -> Bus Creator/4  "Irms Right"
  APPS/1 -> Bus Creator/5  "APPS"
  Steering/1 -> Bus Creator/6  "Steering"
  Differential Toggle/1 -> Bus Creator/7  "Differential Toggle"
  "Regen Enable "/1 -> Bus Creator/8  "Regen Enable"
  Bus Creator/1 -> Bus Selector1/1, Bus Selector3/1, Bus Selector2/1, Bus Selector/1
  Bus Selector/1 -> Power Limiter v3 (open-loop)/2("IDC ")  "<IDC>"
  Bus Selector/2 -> Power Limiter v3 (open-loop)/3(RPM Max)  "<RPM Max>"
  Bus Selector/3 -> Power Limiter v3 (open-loop)/4(Irms Left)  "<Irms Left>"
  Bus Selector/4 -> Power Limiter v3 (open-loop)/5(Irms Right)  "<Irms Right>"
  Bus Selector/5 -> Power Limiter v3 (open-loop)/6(APPS)  "<APPS>"
  Power Limiter v3 (open-loop)/1(Torque Ref PL) -> Electronic Differential/1(Torque Right PL), Electronic Differential/2(Torque Left PL)
  Bus Selector1/1 -> Electronic Differential/3(Steering)  "<Steering>"
  Bus Selector1/2 -> Electronic Differential/4(Differential Toggle)  "<Differential Toggle>"
  Bus Selector2/1 -> Regen/1("IDC ")  "<IDC>"
  Bus Selector2/2 -> Regen/2("Regen Enable ")  "<Regen Enable>"
  Bus Selector3/1 -> Switch2/2  "<Regen Enable>"
  Regen/1("Torque Ref Regen ") -> Right Torque Switch/3, Left Torque Switch/3
  Electronic Differential/1(Torque Right ED) -> Right Torque Switch/1
  Electronic Differential/2(Torque Left ED) -> Left Torque Switch/1
  Power Target in kW1/1 -> Power Limiter v3 (open-loop)/1(Power Target kW)

== system Racing_2019/WannabeCooling ==
  Battery Max Temp : Inport
  LV DCDC Temp : Inport  Port=2
  Compare To Constant20 : simulink/Logic and Bit Operations/Compare To Constant  relop=>=  const=Batt_Temp_High_Threshold  OutDataTypeStr=boolean
  Compare To Constant21 : simulink/Logic and Bit Operations/Compare To Constant  relop=<=  const=Batt_Temp_Low_Threshold  OutDataTypeStr=boolean
  Compare To Constant22 : simulink/Logic and Bit Operations/Compare To Constant  relop=>=  const=LV_DCDC_Temp_High_Threshold  OutDataTypeStr=boolean
  Compare To Constant23 : simulink/Logic and Bit Operations/Compare To Constant  relop=<=  const=LV_DCDC_Temp_Low_Threshold  OutDataTypeStr=boolean
  Constant31 : Constant  Value=Accu_Fans_ON
  Constant32 : Constant  Value=Accu_Fans_Enable
  Constant33 : Constant  Value=0
  Constant34 : Constant  Value=Accu_Fans_PWM  OutDataTypeStr=uint8
  Logical Operator16 : Logic  AllPortsSameDT=off  OutDataTypeStr=boolean
  Logical Operator17 : Logic  Operator=OR  AllPortsSameDT=off  OutDataTypeStr=boolean
  Logical Operator18 : Logic  Operator=OR  AllPortsSameDT=off  OutDataTypeStr=boolean
  Logical Operator19 : Logic  AllPortsSameDT=off  OutDataTypeStr=boolean
  Rate Transition : RateTransition  OutPortSampleTime=0.2
  S-R Flip-Flop5 : simulink_extras/Flip Flops/S-R Flip-Flop  initial_condition=0
  Saturation5 : Saturate  UpperLimit=100  LowerLimit=0
  Switch9 : Switch  Criteria=u2 > Threshold
  Terminator5 : Terminator
  Accu Fans PWM : Outport
  Accu Fans Enable : Outport  Port=2
  wires:
  Compare To Constant23/1 -> Logical Operator19/2
  Switch9/1 -> Accu Fans PWM/1
  Compare To Constant21/1 -> Logical Operator19/1
  Logical Operator18/1 -> S-R Flip-Flop5/1
  LV DCDC Temp/1 -> Rate Transition/1
  Logical Operator19/1 -> S-R Flip-Flop5/2
  Compare To Constant20/1 -> Logical Operator18/1
  Logical Operator17/1 -> Logical Operator16/1
  S-R Flip-Flop5/2 -> Terminator5/1
  Constant33/1 -> Switch9/3
  Constant32/1 -> Logical Operator16/2
  Constant34/1 -> Saturation5/1
  Logical Operator16/1 -> Accu Fans Enable/1, Switch9/2
  S-R Flip-Flop5/1 -> Logical Operator17/2
  Battery Max Temp/1 -> Compare To Constant21/1, Compare To Constant20/1
  Saturation5/1 -> Switch9/1
  Constant31/1 -> Logical Operator17/1
  Compare To Constant22/1 -> Logical Operator18/2
  Rate Transition/1 -> Compare To Constant23/1, Compare To Constant22/1
